simulink library "app_Lib"  (R2015b)
settings: Solver=VariableStepAuto  StartTime=0.0  StopTime=10.0  RelTol=1e-3
settings Model: Creator=kmansour  LastModifiedBy=kmansour

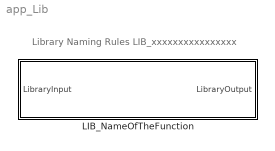
== system app_Lib ==
  note: Library Naming Rules LIB_xxxxxxxxxxxxxxxx
  LIB_NameOfTheFunction : Subsystem

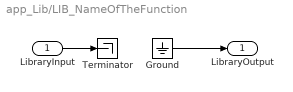
== system app_Lib/LIB_NameOfTheFunction ==
  LibraryInput : Inport
  Ground : Ground
  Terminator : Terminator
  LibraryOutput : Outport
  wires:
  Ground/1 -> LibraryOutput/1
  LibraryInput/1 -> Terminator/1
